simulink model "vehstlin_mdl_callback_mask"  (Simulink 9.0)
settings: Solver=VariableStepAuto  StartTime=0.0  StopTime=10.0  RelTol=1e-3
StopFcn:
  | % Set limits of XY Graph according to simulation
  | block = [bdroot, '/Path'];
  | rto = get_param(block,'RuntimeObject');
  | xmax = rto.InputPort(1).Data;
  | ymax = rto.InputPort(2).Data;
  | set_param(block, 'xmax', num2str(xmax));
  | set_param(block, 'ymax', num2str(ymax));
values from neighbouring files (symbols this model uses):
  A = [a11, 0, a13, 0 ... (first row only)    [vehstlin_sseval.m]
  B = [b11 ... (first row only)    [vehstlin_sseval.m]
  C = [0, 0, 1, 0]    [vehstlin_sseval.m]
  D = 0    [vehstlin_sseval.m]
  v = 20    [vehstlin_param.m]
libraries: simulink x1
settings Model: Creator=hfe2bp  LastModifiedBy=Feri
settings DataIOCC: SaveFormat=Dataset  SaveOutput=off  SignalLogging=off  DSMLogging=off  SaveTime=off
settings OptimizationCC: LifeSpan=auto
settings DebuggingCC: UnderspecifiedInitializationDetection=Simplified  MergeDetectMultiDrivingBlocksExec=error  SFUnexpectedBacktrackingDiag=error  SFNoUnconditionalDefaultTransitionDiag=error  SFExecutionAtInitializationDiag=warning
settings HardwareCC: ProdBitPerPointer=64  ProdBitPerSizeT=64  ProdBitPerPtrDiffT=64  ProdLargestAtomicFloat=Float  ProdIntDivRoundTo=Zero  ProdEndianess=LittleEndian  ProdWordSize=64  ProdHWDeviceType=Intel->x86-64 (Windows64)
settings ModelReferenceCC: PropagateSignalLabelsOutOfModel=on
settings GRTTargetCC: TargetLangStandard=C99 (ISO)
settings ConfigComp: CovMetricSettings=dwe  CovHtmlReporting=off  CovSaveCumulativeToWorkspaceVar=off  CovSaveSingleToWorkspaceVar=off  CovExternalEMLEnable=on

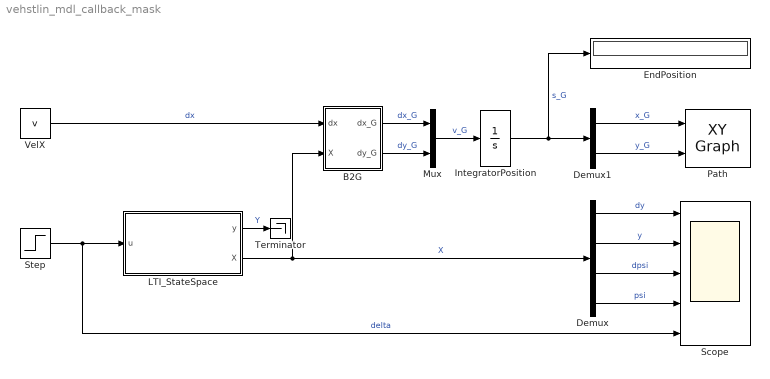
== system vehstlin_mdl_callback_mask ==
  B2G : Subsystem
  Demux : Demux
  Demux1 : Demux  Outputs=2
  EndPosition : Display
  IntegratorPosition : Integrator
  LTI_StateSpace : Subsystem  InitFcn=|  mask(LTI){A=A, B=B, C=C, D=D}
      | vehstlin_param;
      |  [A, B, C, D] = vehstlin_sseval(m, J, v, c_f, c_r, l_f, l_r);
      mask prompts: A "System matrix"; B "Input matrix"; C "Output matrix"; D "Feedthrough matrix"
      mask help: State space representation of a linear time-invariant system.
      mask Display:
      | port_label('input', 1, 'U (input)');
      | port_label('output', 1, 'Y (output)');
      | port_label('output', 2, 'X (state)');
  Mux : Mux  Inputs=2
  Path : simulink/Sinks/XY Graph  xmin=0  xmax=300  ymin=0  ymax=200  st=-1
  Scope : Scope  NumInputPorts=5
  Step : Step  After=1/180*pi  SampleTime=0
  Terminator : Terminator
  VelX : Constant  Value=v
  wires:
  Step/1 -> LTI_StateSpace/1(u), Scope/5  "delta"
  LTI_StateSpace/1(y) -> Terminator/1  "Y"
  Demux/1 -> Scope/1  "dy"
  Demux/2 -> Scope/2  "y"
  Demux/3 -> Scope/3  "dpsi"
  Demux/4 -> Scope/4  "psi"
  VelX/1 -> B2G/1(dx)  "dx"
  B2G/1(dx_G) -> Mux/1  "dx_G"
  B2G/2(dy_G) -> Mux/2  "dy_G"
  Mux/1 -> IntegratorPosition/1  "v_G"
  IntegratorPosition/1 -> EndPosition/1, Demux1/1  "s_G"
  Demux1/1 -> Path/1  "x_G"
  Demux1/2 -> Path/2  "y_G"
  LTI_StateSpace/2(X) -> Demux/1, B2G/2(X)  "X"

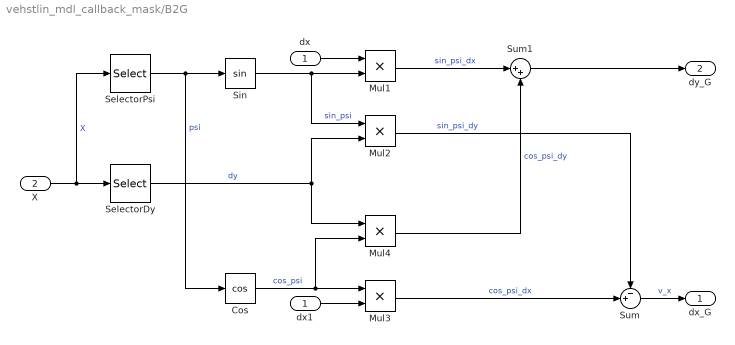
== system vehstlin_mdl_callback_mask/B2G ==
  dx : Inport
  X : Inport  Port=2
  Cos : Trigonometry  Operator=cos
  Mul{1..4} (4 alike) : Product  Inputs=**
  SelectorDy : Selector  InputPortWidth=4  IndexOptions=Index vector (dialog)  Indices=[1]  OutputSizes=1
  SelectorPsi : Selector  InputPortWidth=4  IndexOptions=Index vector (dialog)  Indices=[4]  OutputSizes=1
  Sin : Trigonometry
  Sum : Sum  Inputs=-+|
  Sum1 : Sum  Inputs=|++
  dx1 : InportShadow
  dx_G : Outport
  dy_G : Outport  Port=2
  wires:
  Cos/1 -> Mul4/2, Mul3/1  "cos_psi"
  Sin/1 -> Mul2/1, Mul1/2  "sin_psi"
  SelectorPsi/1 -> Cos/1, Sin/1  "psi"
  X/1 -> SelectorPsi/1, SelectorDy/1  "X"
  SelectorDy/1 -> Mul4/1, Mul2/2  "dy"
  dx/1 -> Mul1/1
  dx1/1 -> Mul3/2
  Mul1/1 -> Sum1/1  "sin_psi_dx"
  Mul2/1 -> Sum/1  "sin_psi_dy"
  Mul4/1 -> Sum1/2  "cos_psi_dy"
  Mul3/1 -> Sum/2  "cos_psi_dx"
  Sum/1 -> dx_G/1  "v_x"
  Sum1/1 -> dy_G/1

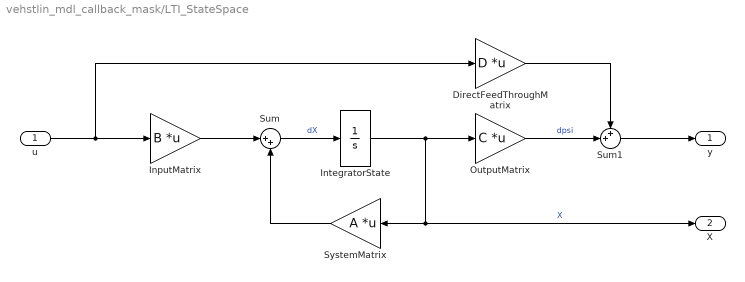
== system vehstlin_mdl_callback_mask/LTI_StateSpace ==
  u : Inport
  DirectFeedThroughMatrix : Gain  Gain=D  Multiplication=Matrix(K*u)
  InputMatrix : Gain  Gain=B  Multiplication=Matrix(K*u)
  IntegratorState : Integrator
  OutputMatrix : Gain  Gain=C  Multiplication=Matrix(K*u)
  Sum : Sum  Inputs=|++
  Sum1 : Sum  Inputs=++|
  SystemMatrix : Gain  Gain=A  Multiplication=Matrix(K*u)
  y : Outport
  X : Outport  Port=2
  wires:
  DirectFeedThroughMatrix/1 -> Sum1/1
  Sum1/1 -> y/1
  OutputMatrix/1 -> Sum1/2  "dpsi"
  u/1 -> DirectFeedThroughMatrix/1, InputMatrix/1
  InputMatrix/1 -> Sum/1
  SystemMatrix/1 -> Sum/2
  IntegratorState/1 -> OutputMatrix/1, SystemMatrix/1, X/1  "X"
  Sum/1 -> IntegratorState/1  "dX"
